simulink model "VU_testSoundTone2"  (Simulink 10.0)
settings: Solver=FixedStepDiscrete  StartTime=0.0  StopTime=inf  FixedStep=0.1  RelTol=1e-3
libraries: lego_nxt_lib x2
settings Model: Creator=jpeytonj  LastModifiedBy=bhisma
settings DataIOCC: LimitDataPoints=on  SignalLoggingSaveFormat=ModelDataLogs
settings OptimizationCC: ExpressionDepthLimit=2147483647
settings DebuggingCC: SolverPrmCheckMsg=warning  FcnCallInpInsideContextMsg=warning  StateNameClashWarn=warning
settings SFSimCC: SimParseCustomCode=off
settings RTWCC: Description=Lego NXT Real-Time Target  SystemTargetFile=lrt.tlc  GenCodeOnly=on  TemplateMakefile=lrt_ecrobot.tmf
settings STFCustomTargetCC: ModelReferenceCompliant=off  GeneratePreprocessorConditionals=Disable all  MatFileLogging=on  CPPClassGenCompliant=on  SystemTargetFile=lrt.tlc
settings GRTTargetCC: ModelReferenceCompliant=off  ParMdlRefBuildCompliant=off  CompOptLevelCompliant=off  ConcurrentExecutionCompliant=off  GeneratePreprocessorConditionals=Disable all  UseToolchainInfoCompliant=off  ExtModeMexFile=noextcomm
settings CustomProperty: DataType=RTWOptions_EnumType_C__Progra~1_MATLAB_R2010a_rtw_c_lrt_lrt_1codeGenType  Value=Integer-only
settings EnumStrPairs: String=Integer-only
settings ConfigComp: CovExternalEMLEnable=off

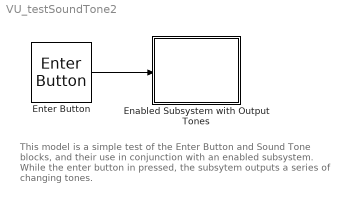
== system VU_testSoundTone2 ==
  note: This model is a simple test of the Enter Button and Sound Tone
      | blocks, and their use in conjunction with an enabled subsystem.
      | While the enter button in pressed, the subsytem outputs a series
      | of changing tones.
  Enabled Subsystem with Output Tones : Subsystem  TreatAsAtomicUnit=on
  Enter Button : lego_nxt_lib/Enter Button  st=0.1
  wires:
  Enter Button/1 -> Enabled Subsystem with Output Tones/Enable

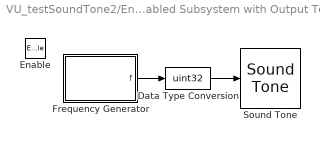
== system VU_testSoundTone2/Enabled Subsystem with Output Tones ==
  Enable : EnablePort
  Data Type Conversion : DataTypeConversion  OutDataTypeStr=uint32
  Frequency Generator : MATLAB Function  TreatAsAtomicUnit=on  SystemSampleTime=0.2
  Sound Tone : lego_nxt_lib/Sound Tone  SystemSampleTime=-1  freqsrc=External  freq=220  volsrc=Internal  vol=50
  wires:
  Frequency Generator/1(f) -> Data Type Conversion/1
  Data Type Conversion/1 -> Sound Tone/1

== matlab function Enabled Subsystem with Output Tones/Frequency Generator ==
  data: f output double
function f = freqGen()

% On each function call, this function will output
% the next frequency from a circular table consisting of the 
% notes [A C# E A] (which define an arpeggio)

% Date:  1 Oct 2010
% Author:  JC Peyton Jones
% Villanova University

% persistent variables for keeping track of state variables
persistent freqTable index

% Initialization
if isempty(freqTable)
    freqTable = [220 277 330 440];  % [A C# E A] ...an arpeggio!
    prevBtn = uint8(0);             % initially unpressed
    index = 0;                      % initially output first freq in table
 end;

% Increment the freqTable index
index= index + 1;
if index > length(freqTable), index = 1; end;
 
% Output the corresponding frequency
f= freqTable(index);
